simulink model "TestForceFilter"  (R2022b)
settings: Solver=FixedStepAuto  StartTime=0.0  StopTime=40  FixedStep=simulator.TimeStep  RelTol=1e-3
settings Model: Creator=At  LastModifiedBy=ateay
settings SolverCC: ConcurrentTasks=on  AlgebraicLoopSolver=TrustRegion  InsertRTBMode=Never (minimum delay)
settings DataIOCC: ReturnWorkspaceOutputs=off
settings DebuggingCC: UnconnectedInputMsg=warning  UnconnectedOutputMsg=warning  UnconnectedLineMsg=warning  SFMachineParentedDataDiag=warning  ArithmeticOperatorsInVariantConditions=warning
settings ModelReferenceCC: EnableRefExpFcnMdlSchedulingChecks=on
settings SFSimCC: SimUseLocalCustomCode=off  CustomCodeUndefinedFunction=UseInterfaceOnly
settings RTWCC: RTWUseLocalCustomCode=off
settings CodeAppCC: StateflowObjectComments=on

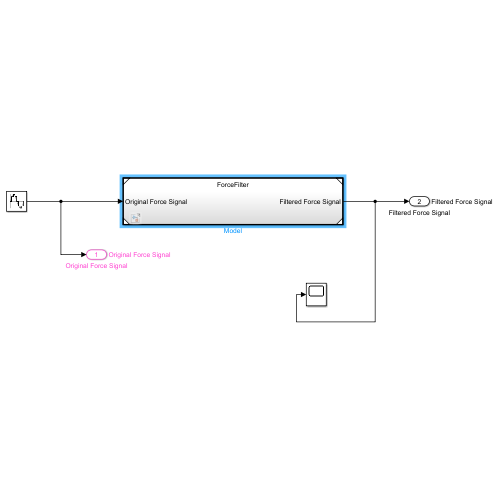
[thumbnail: Simulink's stored preview of the top-level diagram]
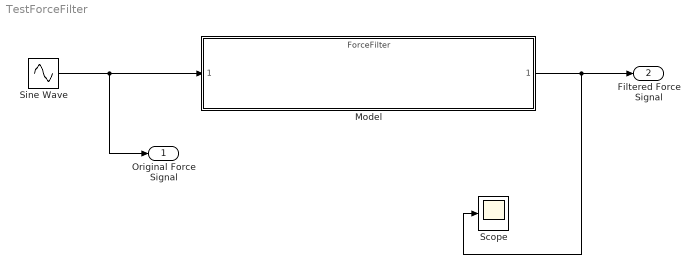
== system TestForceFilter ==
  Model : ModelReference  ModelNameDialog=ForceFilter.slx  SimulationMode=Normal  ModelReferenceVersion=1.2
  Scope : Scope
  Sine Wave : Sin  Frequency=2*pi*6  SampleTime=1/2000
  Original Force Signal : Outport  SignalName=Original Force Signal
  Filtered Force Signal : Outport  Port=2  SignalName=Filtered Force Signal
  wires:
  Model/1 -> Scope/1, Filtered Force Signal/1
  Sine Wave/1 -> Original Force Signal/1, Model/1
